simulink model "poleplace_state_feedback"  (Simulink 7.5)
settings: Solver=ode4  StartTime=0.0  StopTime=10  FixedStep=0.001  RelTol=1e-3
PreLoadFcn:
  | A=[0 1 0;0 0 1;0 -2 -3], B=[0;0;1], C=[10 0 0], K=[4 4 1]
values from neighbouring files (symbols this model uses):
  B = [0; 1],    [poleplace_luenburg_foo_param.m]    (also in poleplace_luenburg_roo_param.m = [0; 0; 1],; poleplace_sfb_luenburg_foo_param.m = [0; 100],; poleplace_sfb_luenburg_roo_param.m = [0; 0; 1],)
  C = [0 1],    [poleplace_luenburg_foo_param.m]    (also in poleplace_luenburg_roo_param.m = [1 0 0],; poleplace_sfb_luenburg_foo_param.m = [1 0],; poleplace_sfb_luenburg_roo_param.m = [1 0 0],)
  K = acker(A, B, p),    [poleplace_sfb_luenburg_foo_param.m]    (also in poleplace_sfb_luenburg_roo_param.m = acker(A, B, pole_ctrl_desired),)
libraries: simulink x1
settings Model: Creator=Huiliang  LastModifiedBy=Dell
settings OptimizationCC: InitFltsAndDblsToZero=on
settings DebuggingCC: SaveWithParameterizedLinksMsg=none  StrictBusMsg=Warning
settings GRTTargetCC: TargetFcnLib=ansi_tfl_tmw.mat

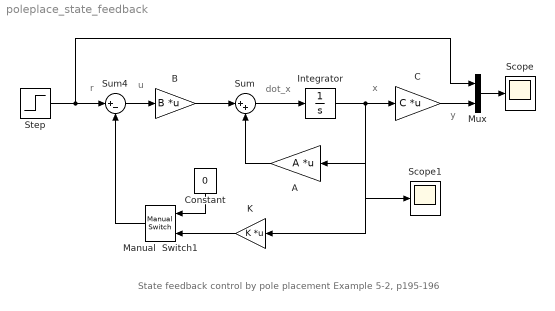
== system poleplace_state_feedback ==
  note: x
  note: dot_x
  note: y
  note: u
  note: r
  note: State feedback control by pole placement
      | Example 5-2, p195-196
  A : Gain  Gain=A  Multiplication=Matrix(K*u)  ParameterDataType=sfix(16)  ParameterScaling=2^0  OutDataType=sfix(16)  OutScaling=2^0
  B : Gain  Gain=B  Multiplication=Matrix(K*u)  ParameterDataType=sfix(16)  ParameterScaling=2^0  OutDataType=sfix(16)  OutScaling=2^0
  C : Gain  Gain=C  Multiplication=Matrix(K*u)  ParameterDataType=sfix(16)  ParameterScaling=2^0  OutDataType=sfix(16)  OutScaling=2^0
  Constant : Constant  Value=0  OutDataType=fixdt(1, 16)  OutScaling=2^0
  Integrator : Integrator  InitialCondition="[0;   0;  0]"
  K : Gain  Gain=K  Multiplication=Matrix(K*u)  ParameterDataType=sfix(16)  ParameterScaling=2^0  OutDataType=sfix(16)  OutScaling=2^0
  Manual  Switch1 : simulink/Signal Routing/Manual Switch  SystemSampleTime=-1  sw=0  action=0  varsize=off
  Mux : Mux  Inputs=2
  Scope : Scope
      settings: TimeRange=10  YMin=0  YMax=3  MaxDataPoints=50000
  Scope1 : Scope
      settings: TimeRange=10  YMin=-0.1  YMax=0.4  MaxDataPoints=50000
  Step : Step  Time=2  SampleTime=0
  Sum : Sum  Inputs=|++  OutDataType=sfix(16)  OutScaling=2^0
  Sum4 : Sum  Inputs=|+-  OutDataType=sfix(16)  OutScaling=2^0
  wires:
  Integrator/1 -> A/1, K/1, Scope1/1, C/1
  Sum/1 -> Integrator/1
  A/1 -> Sum/2
  B/1 -> Sum/1
  Step/1 -> Sum4/1, Mux/1
  Manual  Switch1/1 -> Sum4/2
  Sum4/1 -> B/1
  C/1 -> Mux/2
  Mux/1 -> Scope/1
  K/1 -> Manual  Switch1/2
  Constant/1 -> Manual  Switch1/1
